simulink model "simulation_poursuite_discret"  (Simulink 7.7)
settings: Solver=ode45  StartTime=0  StopTime=5  RelTol=1e-3
values from neighbouring files (symbols this model uses):
  consigne_bf = 1    [PetitGain24V_discret.m]    (also in Vout24V_discret.m)
  pertu_sortie_bf = 1    [PetitGain24V_discret.m]    (also in Vout24V_discret.m)
  Rd = conv(Rd,D)    [PetitGain24V_discret.m]    (also in Vout24V_discret.m)
  Rp = Pc/sum(B)    [PetitGain24V_discret.m]    (also in Vout24V_discret.m)
  Te = 0.0003    [PetitGain24V_discret.m]    (also in Vout24V_discret.m = 0.00035)
undefined symbols (not defined in the file or in its folder): Rn
libraries: cstblocks x1
settings Model: Creator=Nicolas  LastModifiedBy=Nicolas

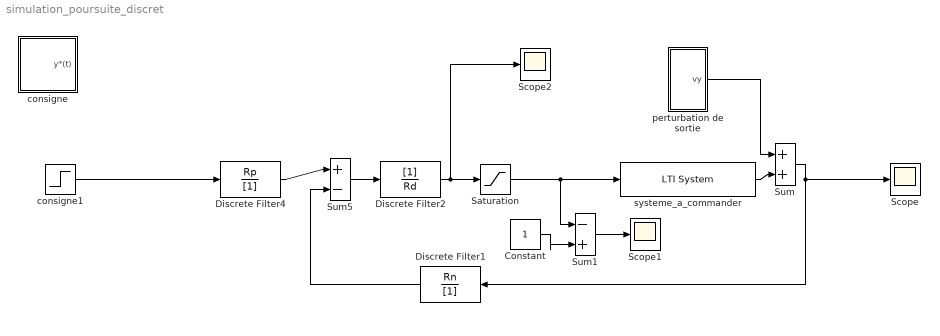
== system simulation_poursuite_discret ==
  Constant : Constant
  Discrete Filter1 : DiscreteFilter  Numerator=Rn  Denominator=[1]  SampleTime=Te
  Discrete Filter2 : DiscreteFilter  Denominator=Rd  SampleTime=Te
  Discrete Filter4 : DiscreteFilter  Numerator=Rp  Denominator=[1]  SampleTime=Te
  Saturation : Saturate  UpperLimit=0.8  LowerLimit=00
  Scope : Scope
      settings: TimeRange=1.5  YMin=-9.999999999999999e+305  YMax=3.5e+306  MaxDataPoints=50000  SampleInput=on  SampleTime=Te
  Scope1 : Scope
      settings: TimeRange=5  YMin=0.1  YMax=1  MaxDataPoints=50000  SampleInput=on  SampleTime=Te
  Scope2 : Scope
      settings: TimeRange=0.1003764115432873  YMin=0.2  YMax=0.2011953551912569  SaveName=ScopeData2  MaxDataPoints=50000  SampleInput=on  SampleTime=Te
  Sum : Sum  Inputs=|++  SampleTime=Te
  Sum1 : Sum  Inputs=|-+  SampleTime=Te
  Sum5 : Sum  Inputs=|+-  SampleTime=Te
  consigne : Subsystem
  consigne1 : Step  After=24  SampleTime=Te
  perturbation de sortie : Subsystem
  systeme_a_commander : cstblocks/LTI System  SystemSampleTime=-1  sys=G_discret  IC=[]
  wires:
  Sum5/1 -> Discrete Filter2/1
  Discrete Filter1/1 -> Sum5/2
  consigne1/1 -> Discrete Filter4/1
  systeme_a_commander/1 -> Sum/2
  Sum/1 -> Scope/1, Discrete Filter1/1
  Discrete Filter2/1 -> Saturation/1, Scope2/1
  Discrete Filter4/1 -> Sum5/1
  Saturation/1 -> systeme_a_commander/1, Sum1/1
  Constant/1 -> Sum1/2
  Sum1/1 -> Scope1/1
  perturbation de sortie/1(vy) -> Sum/1

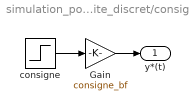
== system simulation_poursuite_discret/consigne ==
  Gain : Gain  Gain=consigne_bf  SampleTime=Te
  consigne : Step  After=24  SampleTime=Te
  y*(t) : Outport
  wires:
  consigne/1 -> Gain/1
  Gain/1 -> y*(t)/1

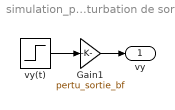
== system simulation_poursuite_discret/perturbation de sortie ==
  Gain1 : Gain  Gain=pertu_sortie_bf
  vy(t) : Step  Time=1.5  SampleTime=0
  vy : Outport
  wires:
  Gain1/1 -> vy/1
  vy(t)/1 -> Gain1/1
